simulink model "pid3_1"  (R2023b)
settings: Solver=VariableStepAuto  StartTime=0.0  StopTime=5  RelTol=1e-3
libraries: simulink x2
settings Model: Creator=Lenovo  LastModifiedBy=21917
settings RTWCC: GPUComputeCapability=5.0

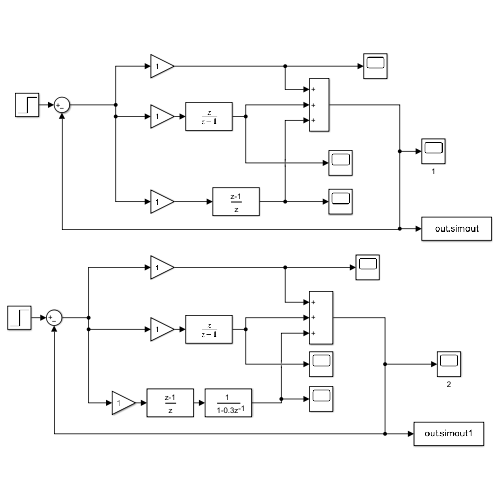
[thumbnail: Simulink's stored preview of the top-level diagram]
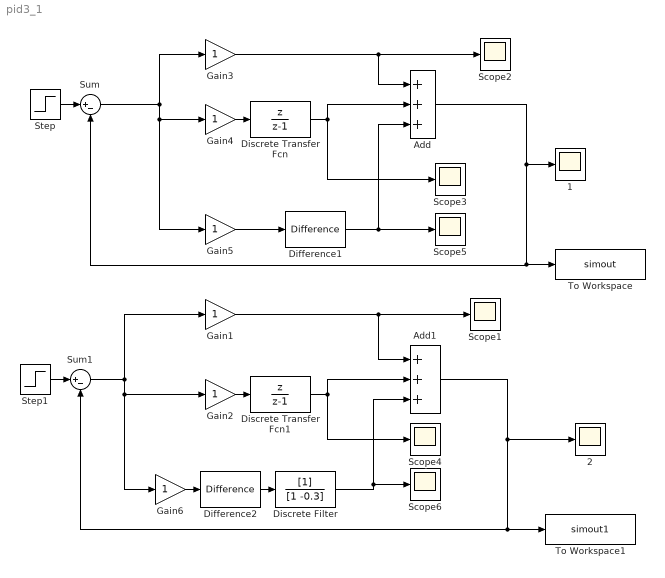
== system pid3_1 ==
  1 : Scope
  2 : Scope
  Add : Sum  Inputs=+++
  Add1 : Sum  Inputs=+++
  Difference1 : simulink/Discrete/Difference  ICPrevInput=0.0  OutMin=[]  OutMax=[]  OutDataType=fixdt(1, 16)  OutScaling=2^-10  DoSatur=off
  Difference2 : simulink/Discrete/Difference  ICPrevInput=0.0  OutMin=[]  OutMax=[]  OutDataType=fixdt(1, 16)  OutScaling=2^-10  DoSatur=off
  Discrete Transfer Fcn : DiscreteTransferFcn  Numerator=[1 0]  Denominator=[1 -1]
  Discrete Transfer Fcn1 : DiscreteTransferFcn  Numerator=[1 0]  Denominator=[1 -1]
  Discrete Filter : DiscreteFilter  Denominator=[1 -0.3]
  Gain{1..6} (6 alike) : Gain
  Scope{1..6} (6 alike) : Scope
  Step : Step  SampleTime=0.1
  Step1 : Step  SampleTime=0.1
  Sum : Sum  Inputs=|+-
  Sum1 : Sum  Inputs=|+-
  To Workspace : ToWorkspace  VariableName=simout  SaveFormat=Timeseries  SampleTime=-1
  To Workspace1 : ToWorkspace  VariableName=simout1  SaveFormat=Timeseries  SampleTime=-1
  wires:
  Gain4/1 -> Discrete Transfer Fcn/1
  Difference1/1 -> Add/3, Scope5/1
  Gain5/1 -> Difference1/1
  Gain3/1 -> Scope2/1, Add/1
  Sum/1 -> Gain3/1, Gain5/1, Gain4/1
  Discrete Transfer Fcn/1 -> Scope3/1, Add/2
  Step/1 -> Sum/1
  Add/1 -> 1/1, To Workspace/1, Sum/2
  Sum1/1 -> Gain1/1, Gain6/1, Gain2/1
  Step1/1 -> Sum1/1
  Add1/1 -> 2/1, To Workspace1/1, Sum1/2
  Gain2/1 -> Discrete Transfer Fcn1/1
  Discrete Transfer Fcn1/1 -> Scope4/1, Add1/2
  Gain6/1 -> Difference2/1
  Gain1/1 -> Add1/1, Scope1/1
  Difference2/1 -> Discrete Filter/1
  Discrete Filter/1 -> Scope6/1, Add1/3
